simulink model "model_cnn"  (R2020a)
settings: Solver=VariableStepAuto  StartTime=0.0  StopTime=1e6/fs  RelTol=1e-3
PreLoadFcn:
  | setup_imports;
  | %dense2_numerictype = fixdt(1,18,10);
  | %conv1_numerictype = fixdt(1,18,21);
InitFcn:
  | % Intermediate signal dimensions
  | input_dim = [1, 2, 128];
  | layer1_dim = hInterConvLayerDims([1,3,1,64],input_dim,1); % dims : [C,H,W]
  | layer2_dim = hInterConvLayerDims([2,3,64,16],layer1_dim,1);% dims : [C,H,W]
  | layer3_dim = [1,128];
  | 
  | % Conv Layer 1 dimensions
  | conv1_dims = struct(...
  |     'input_dim',    input_dim,...       input_dim = C,H,W
  |     'filter_dim',   [1, 3, 1, 64],...  filter_dim = K,J,C,N
  |     'stride',       1,...
  |     'row_output',   3,...
  |     'output_dim',   layer1_dim);
  | 
  | % Conv Layer 2 dimensions
  | conv2_dims = struct(...
  |     'input_dim',    layer1_dim,...      input = C,H.W
  |     'filter_dim',   [2, 3, 64, 16],...  filter_dim = K,J,C,N
  |     'stride',       1,...
  |     'row_output',   2*3*64,...
  |     'output_dim',   layer2_dim);
  | 
  | % Dense Layer 1 dimensions
  | dense1_dims = struct(...
  |     'input_dim',    layer2_dim,...      input = C,H,W
  |     'weight_dim',   [1984, 128],...     weight_dim = H,W
  |     'output_dim',   layer3_dim);
  | 
  | % Load saved weights and input
  | setup_imports;
  | 
  | fs = 128e6;
  | fs_axi = 100e6;
  | R = 32;
values from neighbouring files (symbols this model uses):
  datatypeInput = X_test.numerictype    [setup_imports.m]
  gemm_wconv1 = fi(hInterleaveFilters(Wconv1),1,16)    [setup_imports.m]
  gemm_wconv2 = fi(hInterleaveFilters(Wconv2),1,16)    [setup_imports.m]
  wdense1 = fi(Wdense1,1,16)    [setup_imports.m]
  wdense2 = fi(Wdense2,1,16)    [setup_imports.m]
undefined symbols (not defined in the file or in its folder): ltehdlRAMinitPO2
libraries: hdlsllib x1022, dspsigops x3, dspsrcs4 x2
(part 10 of 23)

== system model_cnn/HDL CNN Model/Dense Layer 1/Dense Layer 1/adder125 ==
  In1 : Inport
  In2 : Inport  Port=2
  In3 : Inport  Port=3
  Data Type Conversion : DataTypeConversion  OutDataTypeStr=datatypeLayer3
  Multiply-Accumulate : hdlsllib/HDL Operations/Multiply-Accumulate  opMode=Streaming - using Number of Samples  initValueSetting=Dialog  initValue=0  initValueSetting2=Dialog  initValue2=0  initValueSetting3=Dialog  initValue3=0  num_samples=1984  RndMeth2=Floor  RndMeth3=Floor  datatype2=Inherit: Inherit via back propagation  datatype3=accumoutdatatype3  validOut=on  endInandOut=on  startOut=on  countOut=on  dim=-1  DoSatur=off  parallel=off
      settings: SourceProductBaseCode=SL
  Terminator : Terminator
  Terminator1 : Terminator
  Terminator2 : Terminator
  dataOut : Outport
  wires:
  Data Type Conversion/1 -> dataOut/1
  ? -> Terminator1/1  "validOut"
  In2/1 -> Multiply-Accumulate/1
  In3/1 -> ?
  Multiply-Accumulate/1 -> Data Type Conversion/1
  ? -> Terminator/1  "countOut"
  In1/1 -> Multiply-Accumulate/2
  ? -> Terminator2/1  "vectorOutValid"

== system model_cnn/HDL CNN Model/Dense Layer 1/Dense Layer 1/adder126 ==
  In1 : Inport
  In2 : Inport  Port=2
  In3 : Inport  Port=3
  Data Type Conversion : DataTypeConversion  OutDataTypeStr=datatypeLayer3
  Multiply-Accumulate : hdlsllib/HDL Operations/Multiply-Accumulate  opMode=Streaming - using Number of Samples  initValueSetting=Dialog  initValue=0  initValueSetting2=Dialog  initValue2=0  initValueSetting3=Dialog  initValue3=0  num_samples=1984  RndMeth2=Floor  RndMeth3=Floor  datatype2=Inherit: Inherit via back propagation  datatype3=accumoutdatatype3  validOut=on  endInandOut=on  startOut=on  countOut=on  dim=-1  DoSatur=off  parallel=off
      settings: SourceProductBaseCode=SL
  Terminator : Terminator
  Terminator1 : Terminator
  Terminator2 : Terminator
  dataOut : Outport
  wires:
  Data Type Conversion/1 -> dataOut/1
  ? -> Terminator1/1  "validOut"
  In2/1 -> Multiply-Accumulate/1
  In3/1 -> ?
  Multiply-Accumulate/1 -> Data Type Conversion/1
  ? -> Terminator/1  "countOut"
  In1/1 -> Multiply-Accumulate/2
  ? -> Terminator2/1  "vectorOutValid"

== system model_cnn/HDL CNN Model/Dense Layer 1/Dense Layer 1/adder127 ==
  In1 : Inport
  In2 : Inport  Port=2
  In3 : Inport  Port=3
  Data Type Conversion : DataTypeConversion  OutDataTypeStr=datatypeLayer3
  Multiply-Accumulate : hdlsllib/HDL Operations/Multiply-Accumulate  opMode=Streaming - using Number of Samples  initValueSetting=Dialog  initValue=0  initValueSetting2=Dialog  initValue2=0  initValueSetting3=Dialog  initValue3=0  num_samples=1984  RndMeth2=Floor  RndMeth3=Floor  datatype2=Inherit: Inherit via back propagation  datatype3=accumoutdatatype3  validOut=on  endInandOut=on  startOut=on  countOut=on  dim=-1  DoSatur=off  parallel=off
      settings: SourceProductBaseCode=SL
  Terminator : Terminator
  Terminator1 : Terminator
  Terminator2 : Terminator
  dataOut : Outport
  wires:
  Data Type Conversion/1 -> dataOut/1
  ? -> Terminator1/1  "validOut"
  In2/1 -> Multiply-Accumulate/1
  In3/1 -> ?
  Multiply-Accumulate/1 -> Data Type Conversion/1
  ? -> Terminator/1  "countOut"
  In1/1 -> Multiply-Accumulate/2
  ? -> Terminator2/1  "vectorOutValid"

== system model_cnn/HDL CNN Model/Dense Layer 1/Dense Layer 1/adder13 ==
  In1 : Inport
  In2 : Inport  Port=2
  In3 : Inport  Port=3
  Data Type Conversion : DataTypeConversion  OutDataTypeStr=datatypeLayer3
  Multiply-Accumulate : hdlsllib/HDL Operations/Multiply-Accumulate  opMode=Streaming - using Number of Samples  initValueSetting=Dialog  initValue=0  initValueSetting2=Dialog  initValue2=0  initValueSetting3=Dialog  initValue3=0  num_samples=1984  RndMeth2=Floor  RndMeth3=Floor  datatype2=Inherit: Inherit via back propagation  datatype3=accumoutdatatype3  validOut=on  endInandOut=on  startOut=on  countOut=on  dim=-1  DoSatur=off  parallel=off
      settings: SourceProductBaseCode=SL
  Terminator : Terminator
  Terminator1 : Terminator
  Terminator2 : Terminator
  dataOut : Outport
  wires:
  Data Type Conversion/1 -> dataOut/1
  ? -> Terminator1/1  "validOut"
  In2/1 -> Multiply-Accumulate/1
  In3/1 -> ?
  Multiply-Accumulate/1 -> Data Type Conversion/1
  ? -> Terminator/1  "countOut"
  In1/1 -> Multiply-Accumulate/2
  ? -> Terminator2/1  "vectorOutValid"

== system model_cnn/HDL CNN Model/Dense Layer 1/Dense Layer 1/adder14 ==
  In1 : Inport
  In2 : Inport  Port=2
  In3 : Inport  Port=3
  Data Type Conversion : DataTypeConversion  OutDataTypeStr=datatypeLayer3
  Multiply-Accumulate : hdlsllib/HDL Operations/Multiply-Accumulate  opMode=Streaming - using Number of Samples  initValueSetting=Dialog  initValue=0  initValueSetting2=Dialog  initValue2=0  initValueSetting3=Dialog  initValue3=0  num_samples=1984  RndMeth2=Floor  RndMeth3=Floor  datatype2=Inherit: Inherit via back propagation  datatype3=accumoutdatatype3  validOut=on  endInandOut=on  startOut=on  countOut=on  dim=-1  DoSatur=off  parallel=off
      settings: SourceProductBaseCode=SL
  Terminator : Terminator
  Terminator1 : Terminator
  Terminator2 : Terminator
  dataOut : Outport
  wires:
  Data Type Conversion/1 -> dataOut/1
  ? -> Terminator1/1  "validOut"
  In2/1 -> Multiply-Accumulate/1
  In3/1 -> ?
  Multiply-Accumulate/1 -> Data Type Conversion/1
  ? -> Terminator/1  "countOut"
  In1/1 -> Multiply-Accumulate/2
  ? -> Terminator2/1  "vectorOutValid"

== system model_cnn/HDL CNN Model/Dense Layer 1/Dense Layer 1/adder15 ==
  In1 : Inport
  In2 : Inport  Port=2
  In3 : Inport  Port=3
  Data Type Conversion : DataTypeConversion  OutDataTypeStr=datatypeLayer3
  Multiply-Accumulate : hdlsllib/HDL Operations/Multiply-Accumulate  opMode=Streaming - using Number of Samples  initValueSetting=Dialog  initValue=0  initValueSetting2=Dialog  initValue2=0  initValueSetting3=Dialog  initValue3=0  num_samples=1984  RndMeth2=Floor  RndMeth3=Floor  datatype2=Inherit: Inherit via back propagation  datatype3=accumoutdatatype3  validOut=on  endInandOut=on  startOut=on  countOut=on  dim=-1  DoSatur=off  parallel=off
      settings: SourceProductBaseCode=SL
  Terminator : Terminator
  Terminator1 : Terminator
  Terminator2 : Terminator
  dataOut : Outport
  wires:
  Data Type Conversion/1 -> dataOut/1
  ? -> Terminator1/1  "validOut"
  In2/1 -> Multiply-Accumulate/1
  In3/1 -> ?
  Multiply-Accumulate/1 -> Data Type Conversion/1
  ? -> Terminator/1  "countOut"
  In1/1 -> Multiply-Accumulate/2
  ? -> Terminator2/1  "vectorOutValid"

== system model_cnn/HDL CNN Model/Dense Layer 1/Dense Layer 1/adder16 ==
  In1 : Inport
  In2 : Inport  Port=2
  In3 : Inport  Port=3
  Data Type Conversion : DataTypeConversion  OutDataTypeStr=datatypeLayer3
  Multiply-Accumulate : hdlsllib/HDL Operations/Multiply-Accumulate  opMode=Streaming - using Number of Samples  initValueSetting=Dialog  initValue=0  initValueSetting2=Dialog  initValue2=0  initValueSetting3=Dialog  initValue3=0  num_samples=1984  RndMeth2=Floor  RndMeth3=Floor  datatype2=Inherit: Inherit via back propagation  datatype3=accumoutdatatype3  validOut=on  endInandOut=on  startOut=on  countOut=on  dim=-1  DoSatur=off  parallel=off
      settings: SourceProductBaseCode=SL
  Terminator : Terminator
  Terminator1 : Terminator
  Terminator2 : Terminator
  dataOut : Outport
  wires:
  Data Type Conversion/1 -> dataOut/1
  ? -> Terminator1/1  "validOut"
  In2/1 -> Multiply-Accumulate/1
  In3/1 -> ?
  Multiply-Accumulate/1 -> Data Type Conversion/1
  ? -> Terminator/1  "countOut"
  In1/1 -> Multiply-Accumulate/2
  ? -> Terminator2/1  "vectorOutValid"

== system model_cnn/HDL CNN Model/Dense Layer 1/Dense Layer 1/adder17 ==
  In1 : Inport
  In2 : Inport  Port=2
  In3 : Inport  Port=3
  Data Type Conversion : DataTypeConversion  OutDataTypeStr=datatypeLayer3
  Multiply-Accumulate : hdlsllib/HDL Operations/Multiply-Accumulate  opMode=Streaming - using Number of Samples  initValueSetting=Dialog  initValue=0  initValueSetting2=Dialog  initValue2=0  initValueSetting3=Dialog  initValue3=0  num_samples=1984  RndMeth2=Floor  RndMeth3=Floor  datatype2=Inherit: Inherit via back propagation  datatype3=accumoutdatatype3  validOut=on  endInandOut=on  startOut=on  countOut=on  dim=-1  DoSatur=off  parallel=off
      settings: SourceProductBaseCode=SL
  Terminator : Terminator
  Terminator1 : Terminator
  Terminator2 : Terminator
  dataOut : Outport
  wires:
  Data Type Conversion/1 -> dataOut/1
  ? -> Terminator1/1  "validOut"
  In2/1 -> Multiply-Accumulate/1
  In3/1 -> ?
  Multiply-Accumulate/1 -> Data Type Conversion/1
  ? -> Terminator/1  "countOut"
  In1/1 -> Multiply-Accumulate/2
  ? -> Terminator2/1  "vectorOutValid"

== system model_cnn/HDL CNN Model/Dense Layer 1/Dense Layer 1/adder18 ==
  In1 : Inport
  In2 : Inport  Port=2
  In3 : Inport  Port=3
  Data Type Conversion : DataTypeConversion  OutDataTypeStr=datatypeLayer3
  Multiply-Accumulate : hdlsllib/HDL Operations/Multiply-Accumulate  opMode=Streaming - using Number of Samples  initValueSetting=Dialog  initValue=0  initValueSetting2=Dialog  initValue2=0  initValueSetting3=Dialog  initValue3=0  num_samples=1984  RndMeth2=Floor  RndMeth3=Floor  datatype2=Inherit: Inherit via back propagation  datatype3=accumoutdatatype3  validOut=on  endInandOut=on  startOut=on  countOut=on  dim=-1  DoSatur=off  parallel=off
      settings: SourceProductBaseCode=SL
  Terminator : Terminator
  Terminator1 : Terminator
  Terminator2 : Terminator
  dataOut : Outport
  wires:
  Data Type Conversion/1 -> dataOut/1
  ? -> Terminator1/1  "validOut"
  In2/1 -> Multiply-Accumulate/1
  In3/1 -> ?
  Multiply-Accumulate/1 -> Data Type Conversion/1
  ? -> Terminator/1  "countOut"
  In1/1 -> Multiply-Accumulate/2
  ? -> Terminator2/1  "vectorOutValid"

== system model_cnn/HDL CNN Model/Dense Layer 1/Dense Layer 1/adder19 ==
  In1 : Inport
  In2 : Inport  Port=2
  In3 : Inport  Port=3
  Data Type Conversion : DataTypeConversion  OutDataTypeStr=datatypeLayer3
  Multiply-Accumulate : hdlsllib/HDL Operations/Multiply-Accumulate  opMode=Streaming - using Number of Samples  initValueSetting=Dialog  initValue=0  initValueSetting2=Dialog  initValue2=0  initValueSetting3=Dialog  initValue3=0  num_samples=1984  RndMeth2=Floor  RndMeth3=Floor  datatype2=Inherit: Inherit via back propagation  datatype3=accumoutdatatype3  validOut=on  endInandOut=on  startOut=on  countOut=on  dim=-1  DoSatur=off  parallel=off
      settings: SourceProductBaseCode=SL
  Terminator : Terminator
  Terminator1 : Terminator
  Terminator2 : Terminator
  dataOut : Outport
  wires:
  Data Type Conversion/1 -> dataOut/1
  ? -> Terminator1/1  "validOut"
  In2/1 -> Multiply-Accumulate/1
  In3/1 -> ?
  Multiply-Accumulate/1 -> Data Type Conversion/1
  ? -> Terminator/1  "countOut"
  In1/1 -> Multiply-Accumulate/2
  ? -> Terminator2/1  "vectorOutValid"

== system model_cnn/HDL CNN Model/Dense Layer 1/Dense Layer 1/adder2 ==
  In1 : Inport
  In2 : Inport  Port=2
  In3 : Inport  Port=3
  Data Type Conversion : DataTypeConversion  OutDataTypeStr=datatypeLayer3
  Multiply-Accumulate : hdlsllib/HDL Operations/Multiply-Accumulate  opMode=Streaming - using Number of Samples  initValueSetting=Dialog  initValue=0  initValueSetting2=Dialog  initValue2=0  initValueSetting3=Dialog  initValue3=0  num_samples=1984  RndMeth2=Floor  RndMeth3=Floor  datatype2=Inherit: Inherit via back propagation  datatype3=accumoutdatatype3  validOut=on  endInandOut=on  startOut=on  countOut=on  dim=-1  DoSatur=off  parallel=off
      settings: SourceProductBaseCode=SL
  Terminator : Terminator
  Terminator1 : Terminator
  Terminator2 : Terminator
  dataOut : Outport
  wires:
  Data Type Conversion/1 -> dataOut/1
  ? -> Terminator1/1  "validOut"
  In2/1 -> Multiply-Accumulate/1
  In3/1 -> ?
  Multiply-Accumulate/1 -> Data Type Conversion/1
  ? -> Terminator/1  "countOut"
  In1/1 -> Multiply-Accumulate/2
  ? -> Terminator2/1  "vectorOutValid"

== system model_cnn/HDL CNN Model/Dense Layer 1/Dense Layer 1/adder20 ==
  In1 : Inport
  In2 : Inport  Port=2
  In3 : Inport  Port=3
  Data Type Conversion : DataTypeConversion  OutDataTypeStr=datatypeLayer3
  Multiply-Accumulate : hdlsllib/HDL Operations/Multiply-Accumulate  opMode=Streaming - using Number of Samples  initValueSetting=Dialog  initValue=0  initValueSetting2=Dialog  initValue2=0  initValueSetting3=Dialog  initValue3=0  num_samples=1984  RndMeth2=Floor  RndMeth3=Floor  datatype2=Inherit: Inherit via back propagation  datatype3=accumoutdatatype3  validOut=on  endInandOut=on  startOut=on  countOut=on  dim=-1  DoSatur=off  parallel=off
      settings: SourceProductBaseCode=SL
  Terminator : Terminator
  Terminator1 : Terminator
  Terminator2 : Terminator
  dataOut : Outport
  wires:
  Data Type Conversion/1 -> dataOut/1
  ? -> Terminator1/1  "validOut"
  In2/1 -> Multiply-Accumulate/1
  In3/1 -> ?
  Multiply-Accumulate/1 -> Data Type Conversion/1
  ? -> Terminator/1  "countOut"
  In1/1 -> Multiply-Accumulate/2
  ? -> Terminator2/1  "vectorOutValid"

== system model_cnn/HDL CNN Model/Dense Layer 1/Dense Layer 1/adder21 ==
  In1 : Inport
  In2 : Inport  Port=2
  In3 : Inport  Port=3
  Data Type Conversion : DataTypeConversion  OutDataTypeStr=datatypeLayer3
  Multiply-Accumulate : hdlsllib/HDL Operations/Multiply-Accumulate  opMode=Streaming - using Number of Samples  initValueSetting=Dialog  initValue=0  initValueSetting2=Dialog  initValue2=0  initValueSetting3=Dialog  initValue3=0  num_samples=1984  RndMeth2=Floor  RndMeth3=Floor  datatype2=Inherit: Inherit via back propagation  datatype3=accumoutdatatype3  validOut=on  endInandOut=on  startOut=on  countOut=on  dim=-1  DoSatur=off  parallel=off
      settings: SourceProductBaseCode=SL
  Terminator : Terminator
  Terminator1 : Terminator
  Terminator2 : Terminator
  dataOut : Outport
  wires:
  Data Type Conversion/1 -> dataOut/1
  ? -> Terminator1/1  "validOut"
  In2/1 -> Multiply-Accumulate/1
  In3/1 -> ?
  Multiply-Accumulate/1 -> Data Type Conversion/1
  ? -> Terminator/1  "countOut"
  In1/1 -> Multiply-Accumulate/2
  ? -> Terminator2/1  "vectorOutValid"

== system model_cnn/HDL CNN Model/Dense Layer 1/Dense Layer 1/adder22 ==
  In1 : Inport
  In2 : Inport  Port=2
  In3 : Inport  Port=3
  Data Type Conversion : DataTypeConversion  OutDataTypeStr=datatypeLayer3
  Multiply-Accumulate : hdlsllib/HDL Operations/Multiply-Accumulate  opMode=Streaming - using Number of Samples  initValueSetting=Dialog  initValue=0  initValueSetting2=Dialog  initValue2=0  initValueSetting3=Dialog  initValue3=0  num_samples=1984  RndMeth2=Floor  RndMeth3=Floor  datatype2=Inherit: Inherit via back propagation  datatype3=accumoutdatatype3  validOut=on  endInandOut=on  startOut=on  countOut=on  dim=-1  DoSatur=off  parallel=off
      settings: SourceProductBaseCode=SL
  Terminator : Terminator
  Terminator1 : Terminator
  Terminator2 : Terminator
  dataOut : Outport
  wires:
  Data Type Conversion/1 -> dataOut/1
  ? -> Terminator1/1  "validOut"
  In2/1 -> Multiply-Accumulate/1
  In3/1 -> ?
  Multiply-Accumulate/1 -> Data Type Conversion/1
  ? -> Terminator/1  "countOut"
  In1/1 -> Multiply-Accumulate/2
  ? -> Terminator2/1  "vectorOutValid"

== system model_cnn/HDL CNN Model/Dense Layer 1/Dense Layer 1/adder23 ==
  In1 : Inport
  In2 : Inport  Port=2
  In3 : Inport  Port=3
  Data Type Conversion : DataTypeConversion  OutDataTypeStr=datatypeLayer3
  Multiply-Accumulate : hdlsllib/HDL Operations/Multiply-Accumulate  opMode=Streaming - using Number of Samples  initValueSetting=Dialog  initValue=0  initValueSetting2=Dialog  initValue2=0  initValueSetting3=Dialog  initValue3=0  num_samples=1984  RndMeth2=Floor  RndMeth3=Floor  datatype2=Inherit: Inherit via back propagation  datatype3=accumoutdatatype3  validOut=on  endInandOut=on  startOut=on  countOut=on  dim=-1  DoSatur=off  parallel=off
      settings: SourceProductBaseCode=SL
  Terminator : Terminator
  Terminator1 : Terminator
  Terminator2 : Terminator
  dataOut : Outport
  wires:
  Data Type Conversion/1 -> dataOut/1
  ? -> Terminator1/1  "validOut"
  In2/1 -> Multiply-Accumulate/1
  In3/1 -> ?
  Multiply-Accumulate/1 -> Data Type Conversion/1
  ? -> Terminator/1  "countOut"
  In1/1 -> Multiply-Accumulate/2
  ? -> Terminator2/1  "vectorOutValid"

== system model_cnn/HDL CNN Model/Dense Layer 1/Dense Layer 1/adder24 ==
  In1 : Inport
  In2 : Inport  Port=2
  In3 : Inport  Port=3
  Data Type Conversion : DataTypeConversion  OutDataTypeStr=datatypeLayer3
  Multiply-Accumulate : hdlsllib/HDL Operations/Multiply-Accumulate  opMode=Streaming - using Number of Samples  initValueSetting=Dialog  initValue=0  initValueSetting2=Dialog  initValue2=0  initValueSetting3=Dialog  initValue3=0  num_samples=1984  RndMeth2=Floor  RndMeth3=Floor  datatype2=Inherit: Inherit via back propagation  datatype3=accumoutdatatype3  validOut=on  endInandOut=on  startOut=on  countOut=on  dim=-1  DoSatur=off  parallel=off
      settings: SourceProductBaseCode=SL
  Terminator : Terminator
  Terminator1 : Terminator
  Terminator2 : Terminator
  dataOut : Outport
  wires:
  Data Type Conversion/1 -> dataOut/1
  ? -> Terminator1/1  "validOut"
  In2/1 -> Multiply-Accumulate/1
  In3/1 -> ?
  Multiply-Accumulate/1 -> Data Type Conversion/1
  ? -> Terminator/1  "countOut"
  In1/1 -> Multiply-Accumulate/2
  ? -> Terminator2/1  "vectorOutValid"

== system model_cnn/HDL CNN Model/Dense Layer 1/Dense Layer 1/adder25 ==
  In1 : Inport
  In2 : Inport  Port=2
  In3 : Inport  Port=3
  Data Type Conversion : DataTypeConversion  OutDataTypeStr=datatypeLayer3
  Multiply-Accumulate : hdlsllib/HDL Operations/Multiply-Accumulate  opMode=Streaming - using Number of Samples  initValueSetting=Dialog  initValue=0  initValueSetting2=Dialog  initValue2=0  initValueSetting3=Dialog  initValue3=0  num_samples=1984  RndMeth2=Floor  RndMeth3=Floor  datatype2=Inherit: Inherit via back propagation  datatype3=accumoutdatatype3  validOut=on  endInandOut=on  startOut=on  countOut=on  dim=-1  DoSatur=off  parallel=off
      settings: SourceProductBaseCode=SL
  Terminator : Terminator
  Terminator1 : Terminator
  Terminator2 : Terminator
  dataOut : Outport
  wires:
  Data Type Conversion/1 -> dataOut/1
  ? -> Terminator1/1  "validOut"
  In2/1 -> Multiply-Accumulate/1
  In3/1 -> ?
  Multiply-Accumulate/1 -> Data Type Conversion/1
  ? -> Terminator/1  "countOut"
  In1/1 -> Multiply-Accumulate/2
  ? -> Terminator2/1  "vectorOutValid"

== system model_cnn/HDL CNN Model/Dense Layer 1/Dense Layer 1/adder26 ==
  In1 : Inport
  In2 : Inport  Port=2
  In3 : Inport  Port=3
  Data Type Conversion : DataTypeConversion  OutDataTypeStr=datatypeLayer3
  Multiply-Accumulate : hdlsllib/HDL Operations/Multiply-Accumulate  opMode=Streaming - using Number of Samples  initValueSetting=Dialog  initValue=0  initValueSetting2=Dialog  initValue2=0  initValueSetting3=Dialog  initValue3=0  num_samples=1984  RndMeth2=Floor  RndMeth3=Floor  datatype2=Inherit: Inherit via back propagation  datatype3=accumoutdatatype3  validOut=on  endInandOut=on  startOut=on  countOut=on  dim=-1  DoSatur=off  parallel=off
      settings: SourceProductBaseCode=SL
  Terminator : Terminator
  Terminator1 : Terminator
  Terminator2 : Terminator
  dataOut : Outport
  wires:
  Data Type Conversion/1 -> dataOut/1
  ? -> Terminator1/1  "validOut"
  In2/1 -> Multiply-Accumulate/1
  In3/1 -> ?
  Multiply-Accumulate/1 -> Data Type Conversion/1
  ? -> Terminator/1  "countOut"
  In1/1 -> Multiply-Accumulate/2
  ? -> Terminator2/1  "vectorOutValid"

== system model_cnn/HDL CNN Model/Dense Layer 1/Dense Layer 1/adder27 ==
  In1 : Inport
  In2 : Inport  Port=2
  In3 : Inport  Port=3
  Data Type Conversion : DataTypeConversion  OutDataTypeStr=datatypeLayer3
  Multiply-Accumulate : hdlsllib/HDL Operations/Multiply-Accumulate  opMode=Streaming - using Number of Samples  initValueSetting=Dialog  initValue=0  initValueSetting2=Dialog  initValue2=0  initValueSetting3=Dialog  initValue3=0  num_samples=1984  RndMeth2=Floor  RndMeth3=Floor  datatype2=Inherit: Inherit via back propagation  datatype3=accumoutdatatype3  validOut=on  endInandOut=on  startOut=on  countOut=on  dim=-1  DoSatur=off  parallel=off
      settings: SourceProductBaseCode=SL
  Terminator : Terminator
  Terminator1 : Terminator
  Terminator2 : Terminator
  dataOut : Outport
  wires:
  Data Type Conversion/1 -> dataOut/1
  ? -> Terminator1/1  "validOut"
  In2/1 -> Multiply-Accumulate/1
  In3/1 -> ?
  Multiply-Accumulate/1 -> Data Type Conversion/1
  ? -> Terminator/1  "countOut"
  In1/1 -> Multiply-Accumulate/2
  ? -> Terminator2/1  "vectorOutValid"

== system model_cnn/HDL CNN Model/Dense Layer 1/Dense Layer 1/adder28 ==
  In1 : Inport
  In2 : Inport  Port=2
  In3 : Inport  Port=3
  Data Type Conversion : DataTypeConversion  OutDataTypeStr=datatypeLayer3
  Multiply-Accumulate : hdlsllib/HDL Operations/Multiply-Accumulate  opMode=Streaming - using Number of Samples  initValueSetting=Dialog  initValue=0  initValueSetting2=Dialog  initValue2=0  initValueSetting3=Dialog  initValue3=0  num_samples=1984  RndMeth2=Floor  RndMeth3=Floor  datatype2=Inherit: Inherit via back propagation  datatype3=accumoutdatatype3  validOut=on  endInandOut=on  startOut=on  countOut=on  dim=-1  DoSatur=off  parallel=off
      settings: SourceProductBaseCode=SL
  Terminator : Terminator
  Terminator1 : Terminator
  Terminator2 : Terminator
  dataOut : Outport
  wires:
  Data Type Conversion/1 -> dataOut/1
  ? -> Terminator1/1  "validOut"
  In2/1 -> Multiply-Accumulate/1
  In3/1 -> ?
  Multiply-Accumulate/1 -> Data Type Conversion/1
  ? -> Terminator/1  "countOut"
  In1/1 -> Multiply-Accumulate/2
  ? -> Terminator2/1  "vectorOutValid"

== system model_cnn/HDL CNN Model/Dense Layer 1/Dense Layer 1/adder29 ==
  In1 : Inport
  In2 : Inport  Port=2
  In3 : Inport  Port=3
  Data Type Conversion : DataTypeConversion  OutDataTypeStr=datatypeLayer3
  Multiply-Accumulate : hdlsllib/HDL Operations/Multiply-Accumulate  opMode=Streaming - using Number of Samples  initValueSetting=Dialog  initValue=0  initValueSetting2=Dialog  initValue2=0  initValueSetting3=Dialog  initValue3=0  num_samples=1984  RndMeth2=Floor  RndMeth3=Floor  datatype2=Inherit: Inherit via back propagation  datatype3=accumoutdatatype3  validOut=on  endInandOut=on  startOut=on  countOut=on  dim=-1  DoSatur=off  parallel=off
      settings: SourceProductBaseCode=SL
  Terminator : Terminator
  Terminator1 : Terminator
  Terminator2 : Terminator
  dataOut : Outport
  wires:
  Data Type Conversion/1 -> dataOut/1
  ? -> Terminator1/1  "validOut"
  In2/1 -> Multiply-Accumulate/1
  In3/1 -> ?
  Multiply-Accumulate/1 -> Data Type Conversion/1
  ? -> Terminator/1  "countOut"
  In1/1 -> Multiply-Accumulate/2
  ? -> Terminator2/1  "vectorOutValid"

== system model_cnn/HDL CNN Model/Dense Layer 1/Dense Layer 1/adder3 ==
  In1 : Inport
  In2 : Inport  Port=2
  In3 : Inport  Port=3
  Data Type Conversion : DataTypeConversion  OutDataTypeStr=datatypeLayer3
  Multiply-Accumulate : hdlsllib/HDL Operations/Multiply-Accumulate  opMode=Streaming - using Number of Samples  initValueSetting=Dialog  initValue=0  initValueSetting2=Dialog  initValue2=0  initValueSetting3=Dialog  initValue3=0  num_samples=1984  RndMeth2=Floor  RndMeth3=Floor  datatype2=Inherit: Inherit via back propagation  datatype3=accumoutdatatype3  validOut=on  endInandOut=on  startOut=on  countOut=on  dim=-1  DoSatur=off  parallel=off
      settings: SourceProductBaseCode=SL
  Terminator : Terminator
  Terminator1 : Terminator
  Terminator2 : Terminator
  dataOut : Outport
  wires:
  Data Type Conversion/1 -> dataOut/1
  ? -> Terminator1/1  "validOut"
  In2/1 -> Multiply-Accumulate/1
  In3/1 -> ?
  Multiply-Accumulate/1 -> Data Type Conversion/1
  ? -> Terminator/1  "countOut"
  In1/1 -> Multiply-Accumulate/2
  ? -> Terminator2/1  "vectorOutValid"

== system model_cnn/HDL CNN Model/Dense Layer 1/Dense Layer 1/adder30 ==
  In1 : Inport
  In2 : Inport  Port=2
  In3 : Inport  Port=3
  Data Type Conversion : DataTypeConversion  OutDataTypeStr=datatypeLayer3
  Multiply-Accumulate : hdlsllib/HDL Operations/Multiply-Accumulate  opMode=Streaming - using Number of Samples  initValueSetting=Dialog  initValue=0  initValueSetting2=Dialog  initValue2=0  initValueSetting3=Dialog  initValue3=0  num_samples=1984  RndMeth2=Floor  RndMeth3=Floor  datatype2=Inherit: Inherit via back propagation  datatype3=accumoutdatatype3  validOut=on  endInandOut=on  startOut=on  countOut=on  dim=-1  DoSatur=off  parallel=off
      settings: SourceProductBaseCode=SL
  Terminator : Terminator
  Terminator1 : Terminator
  Terminator2 : Terminator
  dataOut : Outport
  wires:
  Data Type Conversion/1 -> dataOut/1
  ? -> Terminator1/1  "validOut"
  In2/1 -> Multiply-Accumulate/1
  In3/1 -> ?
  Multiply-Accumulate/1 -> Data Type Conversion/1
  ? -> Terminator/1  "countOut"
  In1/1 -> Multiply-Accumulate/2
  ? -> Terminator2/1  "vectorOutValid"

== system model_cnn/HDL CNN Model/Dense Layer 1/Dense Layer 1/adder31 ==
  In1 : Inport
  In2 : Inport  Port=2
  In3 : Inport  Port=3
  Data Type Conversion : DataTypeConversion  OutDataTypeStr=datatypeLayer3
  Multiply-Accumulate : hdlsllib/HDL Operations/Multiply-Accumulate  opMode=Streaming - using Number of Samples  initValueSetting=Dialog  initValue=0  initValueSetting2=Dialog  initValue2=0  initValueSetting3=Dialog  initValue3=0  num_samples=1984  RndMeth2=Floor  RndMeth3=Floor  datatype2=Inherit: Inherit via back propagation  datatype3=accumoutdatatype3  validOut=on  endInandOut=on  startOut=on  countOut=on  dim=-1  DoSatur=off  parallel=off
      settings: SourceProductBaseCode=SL
  Terminator : Terminator
  Terminator1 : Terminator
  Terminator2 : Terminator
  dataOut : Outport
  wires:
  Data Type Conversion/1 -> dataOut/1
  ? -> Terminator1/1  "validOut"
  In2/1 -> Multiply-Accumulate/1
  In3/1 -> ?
  Multiply-Accumulate/1 -> Data Type Conversion/1
  ? -> Terminator/1  "countOut"
  In1/1 -> Multiply-Accumulate/2
  ? -> Terminator2/1  "vectorOutValid"

== system model_cnn/HDL CNN Model/Dense Layer 1/Dense Layer 1/adder32 ==
  In1 : Inport
  In2 : Inport  Port=2
  In3 : Inport  Port=3
  Data Type Conversion : DataTypeConversion  OutDataTypeStr=datatypeLayer3
  Multiply-Accumulate : hdlsllib/HDL Operations/Multiply-Accumulate  opMode=Streaming - using Number of Samples  initValueSetting=Dialog  initValue=0  initValueSetting2=Dialog  initValue2=0  initValueSetting3=Dialog  initValue3=0  num_samples=1984  RndMeth2=Floor  RndMeth3=Floor  datatype2=Inherit: Inherit via back propagation  datatype3=accumoutdatatype3  validOut=on  endInandOut=on  startOut=on  countOut=on  dim=-1  DoSatur=off  parallel=off
      settings: SourceProductBaseCode=SL
  Terminator : Terminator
  Terminator1 : Terminator
  Terminator2 : Terminator
  dataOut : Outport
  wires:
  Data Type Conversion/1 -> dataOut/1
  ? -> Terminator1/1  "validOut"
  In2/1 -> Multiply-Accumulate/1
  In3/1 -> ?
  Multiply-Accumulate/1 -> Data Type Conversion/1
  ? -> Terminator/1  "countOut"
  In1/1 -> Multiply-Accumulate/2
  ? -> Terminator2/1  "vectorOutValid"

== system model_cnn/HDL CNN Model/Dense Layer 1/Dense Layer 1/adder33 ==
  In1 : Inport
  In2 : Inport  Port=2
  In3 : Inport  Port=3
  Data Type Conversion : DataTypeConversion  OutDataTypeStr=datatypeLayer3
  Multiply-Accumulate : hdlsllib/HDL Operations/Multiply-Accumulate  opMode=Streaming - using Number of Samples  initValueSetting=Dialog  initValue=0  initValueSetting2=Dialog  initValue2=0  initValueSetting3=Dialog  initValue3=0  num_samples=1984  RndMeth2=Floor  RndMeth3=Floor  datatype2=Inherit: Inherit via back propagation  datatype3=accumoutdatatype3  validOut=on  endInandOut=on  startOut=on  countOut=on  dim=-1  DoSatur=off  parallel=off
      settings: SourceProductBaseCode=SL
  Terminator : Terminator
  Terminator1 : Terminator
  Terminator2 : Terminator
  dataOut : Outport
  wires:
  Data Type Conversion/1 -> dataOut/1
  ? -> Terminator1/1  "validOut"
  In2/1 -> Multiply-Accumulate/1
  In3/1 -> ?
  Multiply-Accumulate/1 -> Data Type Conversion/1
  ? -> Terminator/1  "countOut"
  In1/1 -> Multiply-Accumulate/2
  ? -> Terminator2/1  "vectorOutValid"

== system model_cnn/HDL CNN Model/Dense Layer 1/Dense Layer 1/adder34 ==
  In1 : Inport
  In2 : Inport  Port=2
  In3 : Inport  Port=3
  Data Type Conversion : DataTypeConversion  OutDataTypeStr=datatypeLayer3
  Multiply-Accumulate : hdlsllib/HDL Operations/Multiply-Accumulate  opMode=Streaming - using Number of Samples  initValueSetting=Dialog  initValue=0  initValueSetting2=Dialog  initValue2=0  initValueSetting3=Dialog  initValue3=0  num_samples=1984  RndMeth2=Floor  RndMeth3=Floor  datatype2=Inherit: Inherit via back propagation  datatype3=accumoutdatatype3  validOut=on  endInandOut=on  startOut=on  countOut=on  dim=-1  DoSatur=off  parallel=off
      settings: SourceProductBaseCode=SL
  Terminator : Terminator
  Terminator1 : Terminator
  Terminator2 : Terminator
  dataOut : Outport
  wires:
  Data Type Conversion/1 -> dataOut/1
  ? -> Terminator1/1  "validOut"
  In2/1 -> Multiply-Accumulate/1
  In3/1 -> ?
  Multiply-Accumulate/1 -> Data Type Conversion/1
  ? -> Terminator/1  "countOut"
  In1/1 -> Multiply-Accumulate/2
  ? -> Terminator2/1  "vectorOutValid"

== system model_cnn/HDL CNN Model/Dense Layer 1/Dense Layer 1/adder35 ==
  In1 : Inport
  In2 : Inport  Port=2
  In3 : Inport  Port=3
  Data Type Conversion : DataTypeConversion  OutDataTypeStr=datatypeLayer3
  Multiply-Accumulate : hdlsllib/HDL Operations/Multiply-Accumulate  opMode=Streaming - using Number of Samples  initValueSetting=Dialog  initValue=0  initValueSetting2=Dialog  initValue2=0  initValueSetting3=Dialog  initValue3=0  num_samples=1984  RndMeth2=Floor  RndMeth3=Floor  datatype2=Inherit: Inherit via back propagation  datatype3=accumoutdatatype3  validOut=on  endInandOut=on  startOut=on  countOut=on  dim=-1  DoSatur=off  parallel=off
      settings: SourceProductBaseCode=SL
  Terminator : Terminator
  Terminator1 : Terminator
  Terminator2 : Terminator
  dataOut : Outport
  wires:
  Data Type Conversion/1 -> dataOut/1
  ? -> Terminator1/1  "validOut"
  In2/1 -> Multiply-Accumulate/1
  In3/1 -> ?
  Multiply-Accumulate/1 -> Data Type Conversion/1
  ? -> Terminator/1  "countOut"
  In1/1 -> Multiply-Accumulate/2
  ? -> Terminator2/1  "vectorOutValid"

== system model_cnn/HDL CNN Model/Dense Layer 1/Dense Layer 1/adder36 ==
  In1 : Inport
  In2 : Inport  Port=2
  In3 : Inport  Port=3
  Data Type Conversion : DataTypeConversion  OutDataTypeStr=datatypeLayer3
  Multiply-Accumulate : hdlsllib/HDL Operations/Multiply-Accumulate  opMode=Streaming - using Number of Samples  initValueSetting=Dialog  initValue=0  initValueSetting2=Dialog  initValue2=0  initValueSetting3=Dialog  initValue3=0  num_samples=1984  RndMeth2=Floor  RndMeth3=Floor  datatype2=Inherit: Inherit via back propagation  datatype3=accumoutdatatype3  validOut=on  endInandOut=on  startOut=on  countOut=on  dim=-1  DoSatur=off  parallel=off
      settings: SourceProductBaseCode=SL
  Terminator : Terminator
  Terminator1 : Terminator
  Terminator2 : Terminator
  dataOut : Outport
  wires:
  Data Type Conversion/1 -> dataOut/1
  ? -> Terminator1/1  "validOut"
  In2/1 -> Multiply-Accumulate/1
  In3/1 -> ?
  Multiply-Accumulate/1 -> Data Type Conversion/1
  ? -> Terminator/1  "countOut"
  In1/1 -> Multiply-Accumulate/2
  ? -> Terminator2/1  "vectorOutValid"

== system model_cnn/HDL CNN Model/Dense Layer 1/Dense Layer 1/adder37 ==
  In1 : Inport
  In2 : Inport  Port=2
  In3 : Inport  Port=3
  Data Type Conversion : DataTypeConversion  OutDataTypeStr=datatypeLayer3
  Multiply-Accumulate : hdlsllib/HDL Operations/Multiply-Accumulate  opMode=Streaming - using Number of Samples  initValueSetting=Dialog  initValue=0  initValueSetting2=Dialog  initValue2=0  initValueSetting3=Dialog  initValue3=0  num_samples=1984  RndMeth2=Floor  RndMeth3=Floor  datatype2=Inherit: Inherit via back propagation  datatype3=accumoutdatatype3  validOut=on  endInandOut=on  startOut=on  countOut=on  dim=-1  DoSatur=off  parallel=off
      settings: SourceProductBaseCode=SL
  Terminator : Terminator
  Terminator1 : Terminator
  Terminator2 : Terminator
  dataOut : Outport
  wires:
  Data Type Conversion/1 -> dataOut/1
  ? -> Terminator1/1  "validOut"
  In2/1 -> Multiply-Accumulate/1
  In3/1 -> ?
  Multiply-Accumulate/1 -> Data Type Conversion/1
  ? -> Terminator/1  "countOut"
  In1/1 -> Multiply-Accumulate/2
  ? -> Terminator2/1  "vectorOutValid"

== system model_cnn/HDL CNN Model/Dense Layer 1/Dense Layer 1/adder38 ==
  In1 : Inport
  In2 : Inport  Port=2
  In3 : Inport  Port=3
  Data Type Conversion : DataTypeConversion  OutDataTypeStr=datatypeLayer3
  Multiply-Accumulate : hdlsllib/HDL Operations/Multiply-Accumulate  opMode=Streaming - using Number of Samples  initValueSetting=Dialog  initValue=0  initValueSetting2=Dialog  initValue2=0  initValueSetting3=Dialog  initValue3=0  num_samples=1984  RndMeth2=Floor  RndMeth3=Floor  datatype2=Inherit: Inherit via back propagation  datatype3=accumoutdatatype3  validOut=on  endInandOut=on  startOut=on  countOut=on  dim=-1  DoSatur=off  parallel=off
      settings: SourceProductBaseCode=SL
  Terminator : Terminator
  Terminator1 : Terminator
  Terminator2 : Terminator
  dataOut : Outport
  wires:
  Data Type Conversion/1 -> dataOut/1
  ? -> Terminator1/1  "validOut"
  In2/1 -> Multiply-Accumulate/1
  In3/1 -> ?
  Multiply-Accumulate/1 -> Data Type Conversion/1
  ? -> Terminator/1  "countOut"
  In1/1 -> Multiply-Accumulate/2
  ? -> Terminator2/1  "vectorOutValid"

== system model_cnn/HDL CNN Model/Dense Layer 1/Dense Layer 1/adder39 ==
  In1 : Inport
  In2 : Inport  Port=2
  In3 : Inport  Port=3
  Data Type Conversion : DataTypeConversion  OutDataTypeStr=datatypeLayer3
  Multiply-Accumulate : hdlsllib/HDL Operations/Multiply-Accumulate  opMode=Streaming - using Number of Samples  initValueSetting=Dialog  initValue=0  initValueSetting2=Dialog  initValue2=0  initValueSetting3=Dialog  initValue3=0  num_samples=1984  RndMeth2=Floor  RndMeth3=Floor  datatype2=Inherit: Inherit via back propagation  datatype3=accumoutdatatype3  validOut=on  endInandOut=on  startOut=on  countOut=on  dim=-1  DoSatur=off  parallel=off
      settings: SourceProductBaseCode=SL
  Terminator : Terminator
  Terminator1 : Terminator
  Terminator2 : Terminator
  dataOut : Outport
  wires:
  Data Type Conversion/1 -> dataOut/1
  ? -> Terminator1/1  "validOut"
  In2/1 -> Multiply-Accumulate/1
  In3/1 -> ?
  Multiply-Accumulate/1 -> Data Type Conversion/1
  ? -> Terminator/1  "countOut"
  In1/1 -> Multiply-Accumulate/2
  ? -> Terminator2/1  "vectorOutValid"

== system model_cnn/HDL CNN Model/Dense Layer 1/Dense Layer 1/adder4 ==
  In1 : Inport
  In2 : Inport  Port=2
  In3 : Inport  Port=3
  Data Type Conversion : DataTypeConversion  OutDataTypeStr=datatypeLayer3
  Multiply-Accumulate : hdlsllib/HDL Operations/Multiply-Accumulate  opMode=Streaming - using Number of Samples  initValueSetting=Dialog  initValue=0  initValueSetting2=Dialog  initValue2=0  initValueSetting3=Dialog  initValue3=0  num_samples=1984  RndMeth2=Floor  RndMeth3=Floor  datatype2=Inherit: Inherit via back propagation  datatype3=accumoutdatatype3  validOut=on  endInandOut=on  startOut=on  countOut=on  dim=-1  DoSatur=off  parallel=off
      settings: SourceProductBaseCode=SL
  Terminator : Terminator
  Terminator1 : Terminator
  Terminator2 : Terminator
  dataOut : Outport
  wires:
  Data Type Conversion/1 -> dataOut/1
  ? -> Terminator1/1  "validOut"
  In2/1 -> Multiply-Accumulate/1
  In3/1 -> ?
  Multiply-Accumulate/1 -> Data Type Conversion/1
  ? -> Terminator/1  "countOut"
  In1/1 -> Multiply-Accumulate/2
  ? -> Terminator2/1  "vectorOutValid"

== system model_cnn/HDL CNN Model/Dense Layer 1/Dense Layer 1/adder40 ==
  In1 : Inport
  In2 : Inport  Port=2
  In3 : Inport  Port=3
  Data Type Conversion : DataTypeConversion  OutDataTypeStr=datatypeLayer3
  Multiply-Accumulate : hdlsllib/HDL Operations/Multiply-Accumulate  opMode=Streaming - using Number of Samples  initValueSetting=Dialog  initValue=0  initValueSetting2=Dialog  initValue2=0  initValueSetting3=Dialog  initValue3=0  num_samples=1984  RndMeth2=Floor  RndMeth3=Floor  datatype2=Inherit: Inherit via back propagation  datatype3=accumoutdatatype3  validOut=on  endInandOut=on  startOut=on  countOut=on  dim=-1  DoSatur=off  parallel=off
      settings: SourceProductBaseCode=SL
  Terminator : Terminator
  Terminator1 : Terminator
  Terminator2 : Terminator
  dataOut : Outport
  wires:
  Data Type Conversion/1 -> dataOut/1
  ? -> Terminator1/1  "validOut"
  In2/1 -> Multiply-Accumulate/1
  In3/1 -> ?
  Multiply-Accumulate/1 -> Data Type Conversion/1
  ? -> Terminator/1  "countOut"
  In1/1 -> Multiply-Accumulate/2
  ? -> Terminator2/1  "vectorOutValid"

== system model_cnn/HDL CNN Model/Dense Layer 1/Dense Layer 1/adder41 ==
  In1 : Inport
  In2 : Inport  Port=2
  In3 : Inport  Port=3
  Data Type Conversion : DataTypeConversion  OutDataTypeStr=datatypeLayer3
  Multiply-Accumulate : hdlsllib/HDL Operations/Multiply-Accumulate  opMode=Streaming - using Number of Samples  initValueSetting=Dialog  initValue=0  initValueSetting2=Dialog  initValue2=0  initValueSetting3=Dialog  initValue3=0  num_samples=1984  RndMeth2=Floor  RndMeth3=Floor  datatype2=Inherit: Inherit via back propagation  datatype3=accumoutdatatype3  validOut=on  endInandOut=on  startOut=on  countOut=on  dim=-1  DoSatur=off  parallel=off
      settings: SourceProductBaseCode=SL
  Terminator : Terminator
  Terminator1 : Terminator
  Terminator2 : Terminator
  dataOut : Outport
  wires:
  Data Type Conversion/1 -> dataOut/1
  ? -> Terminator1/1  "validOut"
  In2/1 -> Multiply-Accumulate/1
  In3/1 -> ?
  Multiply-Accumulate/1 -> Data Type Conversion/1
  ? -> Terminator/1  "countOut"
  In1/1 -> Multiply-Accumulate/2
  ? -> Terminator2/1  "vectorOutValid"

== system model_cnn/HDL CNN Model/Dense Layer 1/Dense Layer 1/adder42 ==
  In1 : Inport
  In2 : Inport  Port=2
  In3 : Inport  Port=3
  Data Type Conversion : DataTypeConversion  OutDataTypeStr=datatypeLayer3
  Multiply-Accumulate : hdlsllib/HDL Operations/Multiply-Accumulate  opMode=Streaming - using Number of Samples  initValueSetting=Dialog  initValue=0  initValueSetting2=Dialog  initValue2=0  initValueSetting3=Dialog  initValue3=0  num_samples=1984  RndMeth2=Floor  RndMeth3=Floor  datatype2=Inherit: Inherit via back propagation  datatype3=accumoutdatatype3  validOut=on  endInandOut=on  startOut=on  countOut=on  dim=-1  DoSatur=off  parallel=off
      settings: SourceProductBaseCode=SL
  Terminator : Terminator
  Terminator1 : Terminator
  Terminator2 : Terminator
  dataOut : Outport
  wires:
  Data Type Conversion/1 -> dataOut/1
  ? -> Terminator1/1  "validOut"
  In2/1 -> Multiply-Accumulate/1
  In3/1 -> ?
  Multiply-Accumulate/1 -> Data Type Conversion/1
  ? -> Terminator/1  "countOut"
  In1/1 -> Multiply-Accumulate/2
  ? -> Terminator2/1  "vectorOutValid"

== system model_cnn/HDL CNN Model/Dense Layer 1/Dense Layer 1/adder43 ==
  In1 : Inport
  In2 : Inport  Port=2
  In3 : Inport  Port=3
  Data Type Conversion : DataTypeConversion  OutDataTypeStr=datatypeLayer3
  Multiply-Accumulate : hdlsllib/HDL Operations/Multiply-Accumulate  opMode=Streaming - using Number of Samples  initValueSetting=Dialog  initValue=0  initValueSetting2=Dialog  initValue2=0  initValueSetting3=Dialog  initValue3=0  num_samples=1984  RndMeth2=Floor  RndMeth3=Floor  datatype2=Inherit: Inherit via back propagation  datatype3=accumoutdatatype3  validOut=on  endInandOut=on  startOut=on  countOut=on  dim=-1  DoSatur=off  parallel=off
      settings: SourceProductBaseCode=SL
  Terminator : Terminator
  Terminator1 : Terminator
  Terminator2 : Terminator
  dataOut : Outport
  wires:
  Data Type Conversion/1 -> dataOut/1
  ? -> Terminator1/1  "validOut"
  In2/1 -> Multiply-Accumulate/1
  In3/1 -> ?
  Multiply-Accumulate/1 -> Data Type Conversion/1
  ? -> Terminator/1  "countOut"
  In1/1 -> Multiply-Accumulate/2
  ? -> Terminator2/1  "vectorOutValid"

== system model_cnn/HDL CNN Model/Dense Layer 1/Dense Layer 1/adder44 ==
  In1 : Inport
  In2 : Inport  Port=2
  In3 : Inport  Port=3
  Data Type Conversion : DataTypeConversion  OutDataTypeStr=datatypeLayer3
  Multiply-Accumulate : hdlsllib/HDL Operations/Multiply-Accumulate  opMode=Streaming - using Number of Samples  initValueSetting=Dialog  initValue=0  initValueSetting2=Dialog  initValue2=0  initValueSetting3=Dialog  initValue3=0  num_samples=1984  RndMeth2=Floor  RndMeth3=Floor  datatype2=Inherit: Inherit via back propagation  datatype3=accumoutdatatype3  validOut=on  endInandOut=on  startOut=on  countOut=on  dim=-1  DoSatur=off  parallel=off
      settings: SourceProductBaseCode=SL
  Terminator : Terminator
  Terminator1 : Terminator
  Terminator2 : Terminator
  dataOut : Outport
  wires:
  Data Type Conversion/1 -> dataOut/1
  ? -> Terminator1/1  "validOut"
  In2/1 -> Multiply-Accumulate/1
  In3/1 -> ?
  Multiply-Accumulate/1 -> Data Type Conversion/1
  ? -> Terminator/1  "countOut"
  In1/1 -> Multiply-Accumulate/2
  ? -> Terminator2/1  "vectorOutValid"

== system model_cnn/HDL CNN Model/Dense Layer 1/Dense Layer 1/adder45 ==
  In1 : Inport
  In2 : Inport  Port=2
  In3 : Inport  Port=3
  Data Type Conversion : DataTypeConversion  OutDataTypeStr=datatypeLayer3
  Multiply-Accumulate : hdlsllib/HDL Operations/Multiply-Accumulate  opMode=Streaming - using Number of Samples  initValueSetting=Dialog  initValue=0  initValueSetting2=Dialog  initValue2=0  initValueSetting3=Dialog  initValue3=0  num_samples=1984  RndMeth2=Floor  RndMeth3=Floor  datatype2=Inherit: Inherit via back propagation  datatype3=accumoutdatatype3  validOut=on  endInandOut=on  startOut=on  countOut=on  dim=-1  DoSatur=off  parallel=off
      settings: SourceProductBaseCode=SL
  Terminator : Terminator
  Terminator1 : Terminator
  Terminator2 : Terminator
  dataOut : Outport
  wires:
  Data Type Conversion/1 -> dataOut/1
  ? -> Terminator1/1  "validOut"
  In2/1 -> Multiply-Accumulate/1
  In3/1 -> ?
  Multiply-Accumulate/1 -> Data Type Conversion/1
  ? -> Terminator/1  "countOut"
  In1/1 -> Multiply-Accumulate/2
  ? -> Terminator2/1  "vectorOutValid"

== system model_cnn/HDL CNN Model/Dense Layer 1/Dense Layer 1/adder46 ==
  In1 : Inport
  In2 : Inport  Port=2
  In3 : Inport  Port=3
  Data Type Conversion : DataTypeConversion  OutDataTypeStr=datatypeLayer3
  Multiply-Accumulate : hdlsllib/HDL Operations/Multiply-Accumulate  opMode=Streaming - using Number of Samples  initValueSetting=Dialog  initValue=0  initValueSetting2=Dialog  initValue2=0  initValueSetting3=Dialog  initValue3=0  num_samples=1984  RndMeth2=Floor  RndMeth3=Floor  datatype2=Inherit: Inherit via back propagation  datatype3=accumoutdatatype3  validOut=on  endInandOut=on  startOut=on  countOut=on  dim=-1  DoSatur=off  parallel=off
      settings: SourceProductBaseCode=SL
  Terminator : Terminator
  Terminator1 : Terminator
  Terminator2 : Terminator
  dataOut : Outport
  wires:
  Data Type Conversion/1 -> dataOut/1
  ? -> Terminator1/1  "validOut"
  In2/1 -> Multiply-Accumulate/1
  In3/1 -> ?
  Multiply-Accumulate/1 -> Data Type Conversion/1
  ? -> Terminator/1  "countOut"
  In1/1 -> Multiply-Accumulate/2
  ? -> Terminator2/1  "vectorOutValid"

== system model_cnn/HDL CNN Model/Dense Layer 1/Dense Layer 1/adder47 ==
  In1 : Inport
  In2 : Inport  Port=2
  In3 : Inport  Port=3
  Data Type Conversion : DataTypeConversion  OutDataTypeStr=datatypeLayer3
  Multiply-Accumulate : hdlsllib/HDL Operations/Multiply-Accumulate  opMode=Streaming - using Number of Samples  initValueSetting=Dialog  initValue=0  initValueSetting2=Dialog  initValue2=0  initValueSetting3=Dialog  initValue3=0  num_samples=1984  RndMeth2=Floor  RndMeth3=Floor  datatype2=Inherit: Inherit via back propagation  datatype3=accumoutdatatype3  validOut=on  endInandOut=on  startOut=on  countOut=on  dim=-1  DoSatur=off  parallel=off
      settings: SourceProductBaseCode=SL
  Terminator : Terminator
  Terminator1 : Terminator
  Terminator2 : Terminator
  dataOut : Outport
  wires:
  Data Type Conversion/1 -> dataOut/1
  ? -> Terminator1/1  "validOut"
  In2/1 -> Multiply-Accumulate/1
  In3/1 -> ?
  Multiply-Accumulate/1 -> Data Type Conversion/1
  ? -> Terminator/1  "countOut"
  In1/1 -> Multiply-Accumulate/2
  ? -> Terminator2/1  "vectorOutValid"

== system model_cnn/HDL CNN Model/Dense Layer 1/Dense Layer 1/adder48 ==
  In1 : Inport
  In2 : Inport  Port=2
  In3 : Inport  Port=3
  Data Type Conversion : DataTypeConversion  OutDataTypeStr=datatypeLayer3
  Multiply-Accumulate : hdlsllib/HDL Operations/Multiply-Accumulate  opMode=Streaming - using Number of Samples  initValueSetting=Dialog  initValue=0  initValueSetting2=Dialog  initValue2=0  initValueSetting3=Dialog  initValue3=0  num_samples=1984  RndMeth2=Floor  RndMeth3=Floor  datatype2=Inherit: Inherit via back propagation  datatype3=accumoutdatatype3  validOut=on  endInandOut=on  startOut=on  countOut=on  dim=-1  DoSatur=off  parallel=off
      settings: SourceProductBaseCode=SL
  Terminator : Terminator
  Terminator1 : Terminator
  Terminator2 : Terminator
  dataOut : Outport
  wires:
  Data Type Conversion/1 -> dataOut/1
  ? -> Terminator1/1  "validOut"
  In2/1 -> Multiply-Accumulate/1
  In3/1 -> ?
  Multiply-Accumulate/1 -> Data Type Conversion/1
  ? -> Terminator/1  "countOut"
  In1/1 -> Multiply-Accumulate/2
  ? -> Terminator2/1  "vectorOutValid"

== system model_cnn/HDL CNN Model/Dense Layer 1/Dense Layer 1/adder49 ==
  In1 : Inport
  In2 : Inport  Port=2
  In3 : Inport  Port=3
  Data Type Conversion : DataTypeConversion  OutDataTypeStr=datatypeLayer3
  Multiply-Accumulate : hdlsllib/HDL Operations/Multiply-Accumulate  opMode=Streaming - using Number of Samples  initValueSetting=Dialog  initValue=0  initValueSetting2=Dialog  initValue2=0  initValueSetting3=Dialog  initValue3=0  num_samples=1984  RndMeth2=Floor  RndMeth3=Floor  datatype2=Inherit: Inherit via back propagation  datatype3=accumoutdatatype3  validOut=on  endInandOut=on  startOut=on  countOut=on  dim=-1  DoSatur=off  parallel=off
      settings: SourceProductBaseCode=SL
  Terminator : Terminator
  Terminator1 : Terminator
  Terminator2 : Terminator
  dataOut : Outport
  wires:
  Data Type Conversion/1 -> dataOut/1
  ? -> Terminator1/1  "validOut"
  In2/1 -> Multiply-Accumulate/1
  In3/1 -> ?
  Multiply-Accumulate/1 -> Data Type Conversion/1
  ? -> Terminator/1  "countOut"
  In1/1 -> Multiply-Accumulate/2
  ? -> Terminator2/1  "vectorOutValid"

== system model_cnn/HDL CNN Model/Dense Layer 1/Dense Layer 1/adder5 ==
  In1 : Inport
  In2 : Inport  Port=2
  In3 : Inport  Port=3
  Data Type Conversion : DataTypeConversion  OutDataTypeStr=datatypeLayer3
  Multiply-Accumulate : hdlsllib/HDL Operations/Multiply-Accumulate  opMode=Streaming - using Number of Samples  initValueSetting=Dialog  initValue=0  initValueSetting2=Dialog  initValue2=0  initValueSetting3=Dialog  initValue3=0  num_samples=1984  RndMeth2=Floor  RndMeth3=Floor  datatype2=Inherit: Inherit via back propagation  datatype3=accumoutdatatype3  validOut=on  endInandOut=on  startOut=on  countOut=on  dim=-1  DoSatur=off  parallel=off
      settings: SourceProductBaseCode=SL
  Terminator : Terminator
  Terminator1 : Terminator
  Terminator2 : Terminator
  dataOut : Outport
  wires:
  Data Type Conversion/1 -> dataOut/1
  ? -> Terminator1/1  "validOut"
  In2/1 -> Multiply-Accumulate/1
  In3/1 -> ?
  Multiply-Accumulate/1 -> Data Type Conversion/1
  ? -> Terminator/1  "countOut"
  In1/1 -> Multiply-Accumulate/2
  ? -> Terminator2/1  "vectorOutValid"
